simulink model "nonlinear_sim_FG"  (R2015a)
settings: Solver=ode45  StartTime=0.0  StopTime=100  RelTol=1e-3
values from neighbouring files (symbols this model uses):
  cbar = 3.45    [constants.m]
  g = 9.81    [constants.m]
  Iy = 75673.6    [constants.m]
  q_0 = 0    [constants.m]
  theta_0 = 0*(pi/180)    (= 0)    [constants.m]
  u_0 = 135    [constants.m]
  w_0 = 0    [constants.m]
  XE_0 = 0    [constants.m]    (also in controller_design.m)
  ZE_0 = -2000    [constants.m]    (also in controller_design.m)
  zt = 0.15    [constants.m]
undefined symbols (not defined in the file or in its folder): Earth, m, magnitude, WGS84
libraries: aerolibtransform2 x1, aerolibfltsims x1, vrlib x1
settings Model: Creator=vinay  LastModifiedBy=vinay

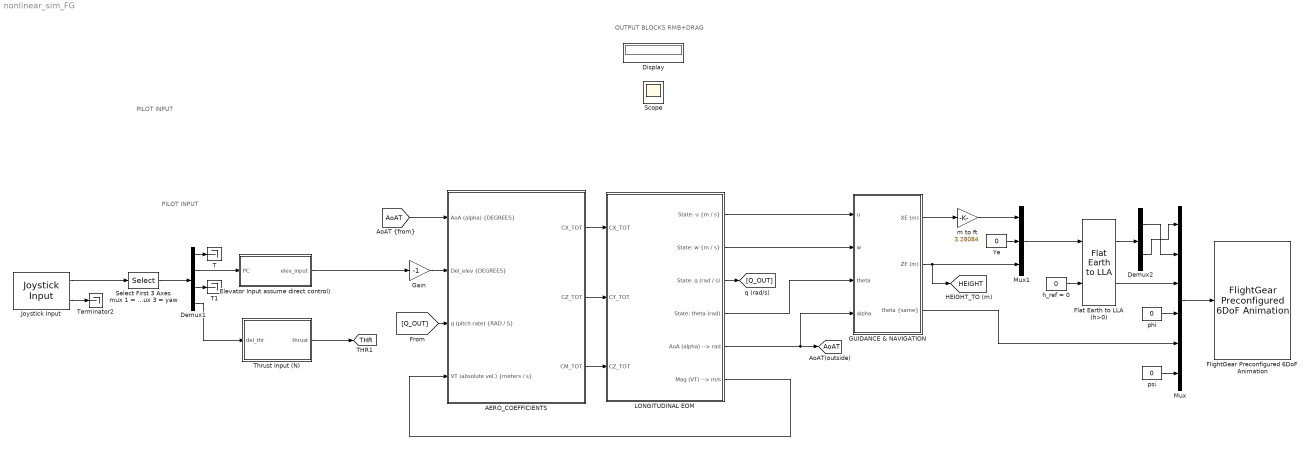
== system nonlinear_sim_FG ==
  note: PILOT INPUT
  note: OUTPUT BLOCKS
      | RMB+DRAG
  note: PILOT INPUT
  "AERO_COEFFICIENTS " : Subsystem
  Demux1 : Demux
  Demux2 : Demux  Outputs=2
  Display : Display
  Elevator Input assume direct control) : Subsystem
  Flat Earth to LLA (h>0) : aerolibtransform2/Flat Earth to LLA  units=Metric (MKS)  ptype=Earth (WGS84)  F=1/298.257223563  R=6378137  LL0=[34.8851654 -117.8323255]  psi=0
  FlightGear Preconfigured 6DoF Animation : aerolibfltsims/FlightGear Preconfigured 6DoF Animation  xFlightGearVersion=v3.0  DestinationIpAddress=127.0.0.1  DestinationPort=5502  SampleTime=1/30
  "GUIDANCE & NAVIGATION " : Subsystem
  Gain : Gain  Gain=-1
  Joystick Input : vrlib/Joystick Input  joyid=1  adjustports=off  forcefeed=off
  LONGITUDINAL EOM : Subsystem
  Mux : Mux  Inputs=6
  Mux1 : Mux  Inputs=3
  Scope : Scope
  Select First 3 Axes mux 1 = roll mux 2 = pitch mux 3 = yaw : Selector  InputPortWidth=8  Indices=[1 2 3 4]
      settings: AttributesFormatString=(Joystick - dependent)
  T : Terminator
  T1 : Terminator
  Terminator2 : Terminator
  Thrust Input (N) : Subsystem
  Ye : Constant  Value=0
  h_ref = 0 : Constant  Value=0
  m to ft : Gain  Gain=3.28084
  phi : Constant  Value=0
  psi : Constant  Value=0
  tag scope: AoAT=global, HEIGHT=global, THR=global
  wires:
  "AERO_COEFFICIENTS "/1(CX_TOT) -> LONGITUDINAL EOM/1(CX_TOT)
  "AERO_COEFFICIENTS "/2(CZ_TOT) -> LONGITUDINAL EOM/2(CY_TOT)
  "AERO_COEFFICIENTS "/3(CM_TOT) -> LONGITUDINAL EOM/3(CZ_TOT)
  [AoAT] -> "AERO_COEFFICIENTS "/1("AoA (alpha) {DEGREES}")
  LONGITUDINAL EOM/6(Mag (VT) --> m/s) -> "AERO_COEFFICIENTS "/4("VT (absolute vel.) {meters / s}")
  Elevator Input assume direct control)/1(elev_input) -> Gain/1
  LONGITUDINAL EOM/5(AoA (alpha) --> rad) -> [AoAT], "GUIDANCE & NAVIGATION "/4(alpha)
  LONGITUDINAL EOM/3(State: q (rad / s)) -> [Q_OUT]
  [Q_OUT] -> "AERO_COEFFICIENTS "/3("q (pitch rate) {RAD / S}")
  LONGITUDINAL EOM/1("State: u {m / s}") -> "GUIDANCE & NAVIGATION "/1(u)
  LONGITUDINAL EOM/2("State: w {m / s}") -> "GUIDANCE & NAVIGATION "/2(w)
  LONGITUDINAL EOM/4(State: theta (rad)) -> "GUIDANCE & NAVIGATION "/3(theta)
  "GUIDANCE & NAVIGATION "/2(ZE (m)) -> Mux1/3, [HEIGHT]
  Demux1/3 -> T1/1
  Select First 3 Axes mux 1 = roll mux 2 = pitch mux 3 = yaw/1 -> Demux1/1
  Demux1/2 -> Elevator Input assume direct control)/1(PC)
  Joystick Input/1 -> Select First 3 Axes mux 1 = roll mux 2 = pitch mux 3 = yaw/1
  Demux1/1 -> T/1
  Joystick Input/2 -> Terminator2/1
  Mux/1 -> FlightGear Preconfigured 6DoF Animation/1
  phi/1 -> Mux/4
  psi/1 -> Mux/6
  "GUIDANCE & NAVIGATION "/1(XE (m)) -> m to ft/1
  Ye/1 -> Mux1/2
  Mux1/1 -> Flat Earth to LLA (h>0)/1
  h_ref = 0/1 -> Flat Earth to LLA (h>0)/2
  Flat Earth to LLA (h>0)/1 -> Demux2/1
  Flat Earth to LLA (h>0)/2 -> Mux/3
  Demux2/1 -> Mux/2
  "GUIDANCE & NAVIGATION "/3("theta {same}") -> Mux/5
  Demux2/2 -> Mux/1
  Gain/1 -> "AERO_COEFFICIENTS "/2("Del_elev {DEGREES}")
  Demux1/4 -> Thrust Input (N)/1(del_thr)
  Thrust Input (N)/1(thrust) -> [THR]
  m to ft/1 -> Mux1/1

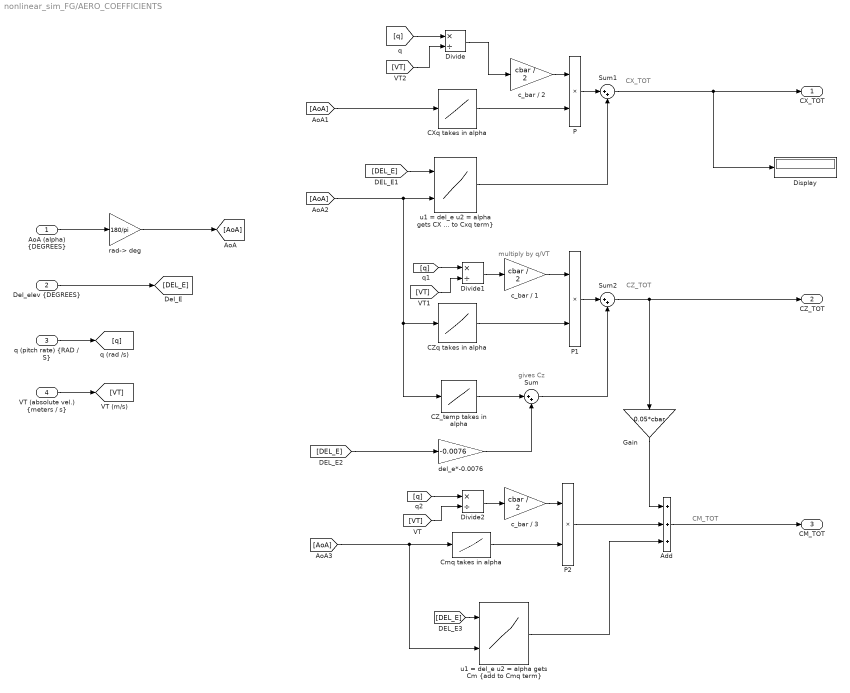
== system nonlinear_sim_FG/AERO_COEFFICIENTS  ==
  note: multiply by q/VT
  note: CM_TOT
  note: CX_TOT
  note: gives Cz
  note: CZ_TOT
  "AoA (alpha) {DEGREES}" : Inport
  "Del_elev {DEGREES}" : Inport  Port=2
  "q (pitch rate) {RAD / S}" : Inport  Port=3
  "VT (absolute vel.) {meters / s}" : Inport  Port=4
  Add : Sum  Inputs=+++
  CXq takes in alpha : Lookup_n-D  NumberOfTableDimensions=1  BreakpointsForDimension1=[-10,-5,0,5,10,15,20,25,30,35,40,45]  BreakpointsForDimension1Min=[-10]  BreakpointsForDimension1Max=[10]  Table=[-.267,.110,.308,1.34,2.08,2.91,2.76,2.05,1.5,1.49,1.83,1.21]  InternalRulePriority=Speed  OutMin=[-1.000]  OutMax=[1.000]  RndMeth=Simplest  InputSameDT=on
  CZ_temp takes in alpha : Lookup_n-D  NumberOfTableDimensions=1  BreakpointsForDimension1=[-10,-5,0,5,10,15,20,25,30,35,40,45]  BreakpointsForDimension1Min=[-10]  BreakpointsForDimension1Max=[10]  Table=[.770, .241, -.100, -.416, -.731, -1.053, -1.366, -1.646, -1.917, -2.120, -2.248, -2.229]  InternalRulePriority=Speed  OutMin=[-1.000]  OutMax=[1.000]  RndMeth=Simplest  InputSameDT=on
  CZq takes in alpha : Lookup_n-D  NumberOfTableDimensions=1  BreakpointsForDimension1=[-10,-5,0,5,10,15,20,25,30,35,40,45]  BreakpointsForDimension1Min=[-10]  BreakpointsForDimension1Max=[10]  Table="[-8.8, -25.8, -28.9, -31.4, -31.2, -30.7, -27.7, -28.2,   -29, -29.8, -38.3, -35.3]"  InternalRulePriority=Speed  OutMin=[-1.000]  OutMax=[1.000]  RndMeth=Simplest  InputSameDT=on
  Cmq takes in alpha : Lookup_n-D  NumberOfTableDimensions=1  BreakpointsForDimension1=[-10,-5,0,5,10,15,20,25,30,35,40,45]  BreakpointsForDimension1Min=[-10]  BreakpointsForDimension1Max=[10]  Table="[-7.21,  -.54, -5.23, -5.26, -6.11, -6.64, -5.69,    -6,  -6.2,  -6.4,  -6.6,    -6]"  InternalRulePriority=Speed  OutMin=[-1.000]  OutMax=[1.000]  RndMeth=Simplest  InputSameDT=on
  Display : Display
  Divide : Product  Inputs=*/
  Divide1 : Product  Inputs=*/
  Divide2 : Product  Inputs=*/
  Gain : Gain  Gain=0.05*cbar
  P : Product
  P1 : Product
  P2 : Product
  Sum : Sum  Inputs=|++
  Sum1 : Sum  Inputs=|++
  Sum2 : Sum  Inputs=|++
  c_bar / 1 : Gain  Gain=cbar / 2
  c_bar / 2 : Gain  Gain=cbar / 2
  c_bar / 3 : Gain  Gain=cbar / 2
  del_e*-0.0076 : Gain  Gain=-0.0076
  rad-> deg : Gain  Gain=180/pi
  "u1 = del_e u2 = alpha gets CX {add to Cxq term}" : Lookup_n-D  BreakpointsForDimension1=[-25 -12.5 0 12.5 25]  BreakpointsForDimension2=[-10 -5 0 5 10 15 20 25 30 35 40 45]  IndexSearchMethod=Evenly spaced points  Table="[-.083, -.073, -.076, -.072, -.046, .012, .024, .025, .043, .053, .047, .040; -.040, -.038, -.039, -.025,  .006, .062, .087, .085, .100, .110, .104, .091;-.022, -.020, -.021, -.004,  .032, .094, .128, .130, .154, .161, .155, .138; -.048, -.038, -.040, -.021,  .016, .083, .127, .137, .162, .177, .179, .167; -.099, -.081, -.081, -.063, -.025, .044, .097, .113, .145, .167, .174, .166]"  InternalRulePriority=Speed  RndMeth=Simplest  InputSameDT=on
  "u1 = del_e u2 = alpha gets Cm {add to Cmq term}" : Lookup_n-D  BreakpointsForDimension1=[-25 -12.5 0 12.5 25]  BreakpointsForDimension2=[-10 -5 0 5 10 15 20 25 30 35 40 45]  IndexSearchMethod=Evenly spaced points  Table="[.205,  .168,  .186,  .196,  .213,  .251,  .245,  .238,  .252,  .231,  .198,  .192; .081,  .077,  .107,  .110,  .110,  .141,  .127,  .119,  .133,  .108,  .081,  .093; -.046, -.020, -.009, -.005, -.006,  .010,  .006, -.001,  .014,   0.0, -.013,  .032; -.174, -.145, -.121, -.127, -.129, -.102, -.097, -.113, -.087, -.084, -.069, -.006; -.259, -.202, -.184, -.193, -.199, -.150, -.160, -.167, -.104, -.076, -.041, -.005]"  InternalRulePriority=Speed  RndMeth=Simplest  InputSameDT=on
  CX_TOT : Outport
  CZ_TOT : Outport  Port=2
  CM_TOT : Outport  Port=3
  wires:
  P2/1 -> Add/2
  "q (pitch rate) {RAD / S}"/1 -> [q]
  Cmq takes in alpha/1 -> P2/2
  Divide2/1 -> c_bar / 3/1
  Add/1 -> CM_TOT/1
  [VT] -> Divide/2
  P1/1 -> Sum2/1
  Sum/1 -> Sum2/2
  CZq takes in alpha/1 -> P1/2
  c_bar / 1/1 -> P1/1
  Sum2/1 -> CZ_TOT/1, Gain/1
  [VT] -> Divide1/2
  del_e*-0.0076/1 -> Sum/2
  CZ_temp takes in alpha/1 -> Sum/1
  P/1 -> Sum1/1
  c_bar / 3/1 -> P2/1
  "u1 = del_e u2 = alpha gets Cm {add to Cmq term}"/1 -> Add/3
  [q] -> Divide1/1
  [DEL_E] -> "u1 = del_e u2 = alpha gets Cm {add to Cmq term}"/1
  "u1 = del_e u2 = alpha gets CX {add to Cxq term}"/1 -> Sum1/2
  CXq takes in alpha/1 -> P/2
  Sum1/1 -> Display/1, CX_TOT/1
  c_bar / 2/1 -> P/1
  "VT (absolute vel.) {meters / s}"/1 -> [VT]
  [DEL_E] -> del_e*-0.0076/1
  [AoA] -> "u1 = del_e u2 = alpha gets CX {add to Cxq term}"/2, CZ_temp takes in alpha/1, CZq takes in alpha/1
  [DEL_E] -> "u1 = del_e u2 = alpha gets CX {add to Cxq term}"/1
  Gain/1 -> Add/1
  "AoA (alpha) {DEGREES}"/1 -> rad-> deg/1
  Divide1/1 -> c_bar / 1/1
  [AoA] -> "u1 = del_e u2 = alpha gets Cm {add to Cmq term}"/2, Cmq takes in alpha/1
  [q] -> Divide/1
  [VT] -> Divide2/2
  Divide/1 -> c_bar / 2/1
  [q] -> Divide2/1
  [AoA] -> CXq takes in alpha/1
  rad-> deg/1 -> [AoA]
  "Del_elev {DEGREES}"/1 -> [DEL_E]

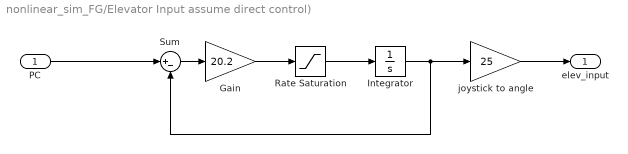
== system nonlinear_sim_FG/Elevator Input assume direct control) ==
  PC : Inport
  Gain : Gain  Gain=20.2  SaturateOnIntegerOverflow=on  OutDataTypeStr=Inherit: Same as input  ParamDataTypeStr=Inherit: Same as input
  "Integrator " : Integrator  InitialCondition=-2.4607  UpperSaturationLimit=25  LowerSaturationLimit=-25
  Rate Saturation : Saturate  UpperLimit=60  LowerLimit=-60
  Sum : Sum  Inputs=|+-  SaturateOnIntegerOverflow=on  InputSameDT=on  OutDataTypeStr=Inherit: Same as first input
  joystick to angle : Gain  Gain=25  SaturateOnIntegerOverflow=on  OutDataTypeStr=Inherit: Same as input  ParamDataTypeStr=Inherit: Same as input
  elev_input : Outport
  wires:
  PC/1 -> Sum/1
  Sum/1 -> Gain/1
  Gain/1 -> Rate Saturation/1
  Rate Saturation/1 -> "Integrator "/1
  "Integrator "/1 -> joystick to angle/1, Sum/2
  joystick to angle/1 -> elev_input/1

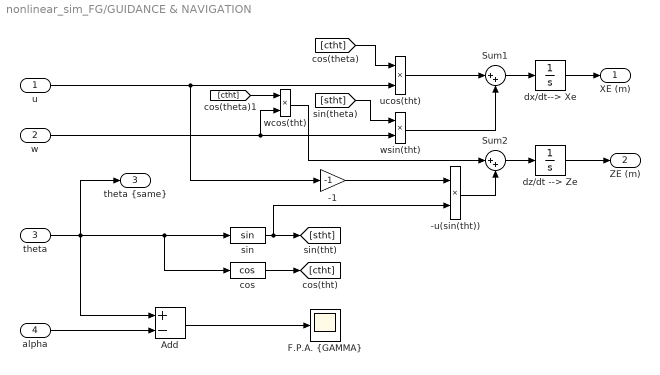
== system nonlinear_sim_FG/GUIDANCE & NAVIGATION  ==
  u : Inport
  w : Inport  Port=2
  theta : Inport  Port=3
  alpha : Inport  Port=4
  -1 : Gain  Gain=-1
  -u(sin(tht)) : Product
  Add : Sum  Inputs=+-
  "F.P.A. {GAMMA}" : Scope
      settings: SaveName=ScopeData2
  Sum1 : Sum  Inputs=|++
  Sum2 : Sum  Inputs=|++
  cos : Trigonometry  Operator=cos
  dx/dt--> Xe : Integrator  InitialCondition=XE_0
  dz/dt --> Ze : Integrator  InitialCondition=ZE_0
  sin : Trigonometry
  ucos(tht) : Product
  wcos(tht) : Product
  wsin(tht) : Product
  XE (m) : Outport
  ZE (m) : Outport  Port=2
  "theta {same}" : Outport  Port=3
  wires:
  [stht] -> wsin(tht)/1
  wsin(tht)/1 -> Sum1/2
  u/1 -> ucos(tht)/2, -1/1
  w/1 -> wcos(tht)/2, wsin(tht)/2
  theta/1 -> "theta {same}"/1, Add/1, cos/1, sin/1
  dx/dt--> Xe/1 -> XE (m)/1
  ucos(tht)/1 -> Sum1/1
  dz/dt --> Ze/1 -> ZE (m)/1
  Sum1/1 -> dx/dt--> Xe/1
  Sum2/1 -> dz/dt --> Ze/1
  cos/1 -> [ctht]
  sin/1 -> -u(sin(tht))/2, [stht]
  wcos(tht)/1 -> Sum2/1
  [ctht] -> wcos(tht)/1
  -1/1 -> -u(sin(tht))/1
  [ctht] -> ucos(tht)/1
  -u(sin(tht))/1 -> Sum2/2
  alpha/1 -> Add/2
  Add/1 -> "F.P.A. {GAMMA}"/1

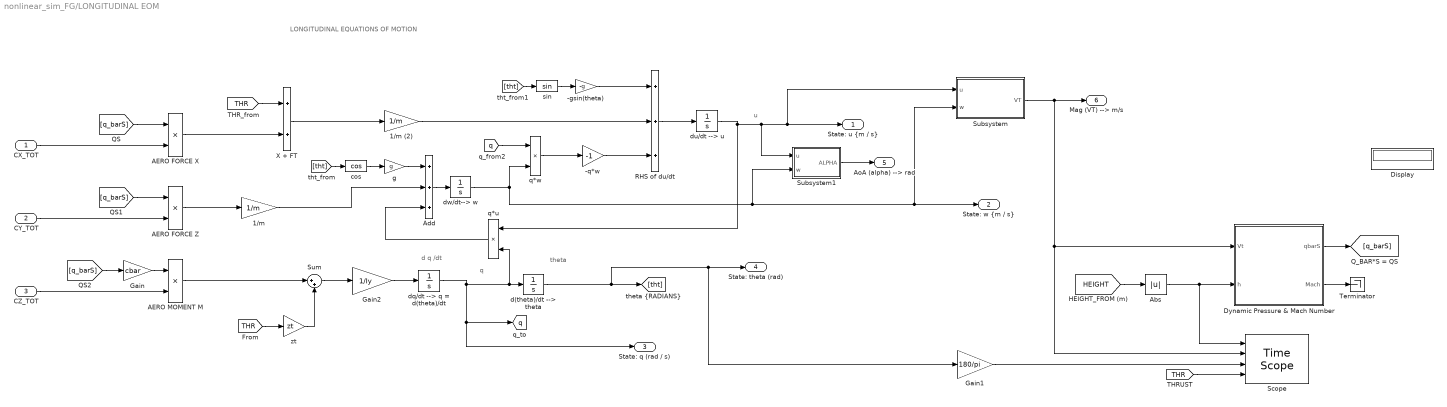
== system nonlinear_sim_FG/LONGITUDINAL EOM ==
  note: LONGITUDINAL EQUATIONS OF MOTION
  note: u
  note: theta
  note: q
  note: d q /dt
  CX_TOT : Inport
  CY_TOT : Inport  Port=2
  CZ_TOT : Inport  Port=3
  -gsin(theta) : Gain  Gain=-g
  -q*w : Gain  Gain=-1
  1/m : Gain  Gain=1/m
  1/m (2) : Gain  Gain=1/m
  AERO FORCE X : Product
  AERO FORCE Z : Product
  AERO MOMENT M : Product
  Abs : Abs
  Add : Sum  Inputs=+++
  Display : Display
  Dynamic Pressure & Mach Number : MATLAB Function  TreatAsAtomicUnit=on
  Gain : Gain  Gain=cbar
  Gain1 : Gain  Gain=180/pi
  Gain2 : Gain  Gain=1/Iy
  RHS of du/dt : Sum  Inputs=+++
  Scope : TimeScope  NumInputPorts=4
  Subsystem : Subsystem
  Subsystem1 : Subsystem
  Sum : Sum  Inputs=|++
  Terminator : Terminator
  X + FT : Sum
  cos : Trigonometry  Operator=cos
  d(theta)/dt --> theta : Integrator  InitialCondition=theta_0
  dq/dt --> q = d(theta)/dt : Integrator  InitialCondition=q_0
  du/dt --> u : Integrator  InitialCondition=u_0  LimitOutput=on  LowerSaturationLimit=0
  dw/dt--> w : Integrator  InitialCondition=w_0
  g : Gain  Gain=g
  q*u : Product
  q*w : Product
  sin : Trigonometry
  zt : Gain  Gain=zt
  "State: u {m / s}" : Outport
  "State: w {m / s}" : Outport  Port=2
  State: q (rad / s) : Outport  Port=3
  State: theta (rad) : Outport  Port=4
  AoA (alpha) --> rad : Outport  Port=5
  Mag (VT) --> m/s : Outport  Port=6
  tag scope: q=global
  wires:
  [THR] -> X + FT/1
  q*w/1 -> -q*w/1
  zt/1 -> Sum/2
  Gain2/1 -> dq/dt --> q = d(theta)/dt/1
  dq/dt --> q = d(theta)/dt/1 -> State: q (rad / s)/1, [q], q*u/2, d(theta)/dt --> theta/1
  -gsin(theta)/1 -> RHS of du/dt/1
  [q] -> q*w/1
  1/m/1 -> Add/2
  AERO FORCE X/1 -> X + FT/2
  AERO MOMENT M/1 -> Sum/1
  [THR] -> zt/1
  [tht] -> sin/1
  sin/1 -> -gsin(theta)/1
  CY_TOT/1 -> AERO FORCE Z/2
  [q_barS] -> AERO FORCE Z/1
  CX_TOT/1 -> AERO FORCE X/2
  [q_barS] -> AERO FORCE X/1
  CZ_TOT/1 -> AERO MOMENT M/2
  [q_barS] -> Gain/1
  Gain/1 -> AERO MOMENT M/1
  d(theta)/dt --> theta/1 -> Gain1/1, State: theta (rad)/1, [tht]
  Sum/1 -> Gain2/1
  AERO FORCE Z/1 -> 1/m/1
  g/1 -> Add/1
  Add/1 -> dw/dt--> w/1
  cos/1 -> g/1
  q*u/1 -> Add/3
  [tht] -> cos/1
  RHS of du/dt/1 -> du/dt --> u/1
  1/m (2)/1 -> RHS of du/dt/2
  X + FT/1 -> 1/m (2)/1
  -q*w/1 -> RHS of du/dt/3
  du/dt --> u/1 -> Subsystem1/1(u), Subsystem/1(u), "State: u {m / s}"/1, q*u/1
  dw/dt--> w/1 -> Subsystem1/2(w), Subsystem/2(w), "State: w {m / s}"/1, q*w/2
  Dynamic Pressure & Mach Number/1(qbarS) -> [q_barS]
  [HEIGHT] -> Abs/1
  Dynamic Pressure & Mach Number/2(Mach) -> Terminator/1
  Subsystem/1(VT) -> Scope/2, Dynamic Pressure & Mach Number/1(Vt), Mag (VT) --> m/s/1
  Subsystem1/1(ALPHA) -> AoA (alpha) --> rad/1
  Abs/1 -> Scope/1, Dynamic Pressure & Mach Number/2(h)
  Gain1/1 -> Scope/3
  [THR] -> Scope/4

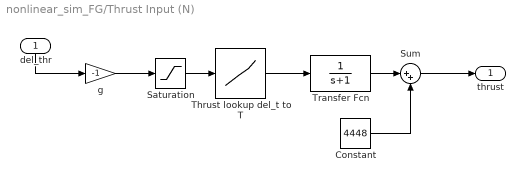
== system nonlinear_sim_FG/Thrust Input (N) ==
  del_thr : Inport
  Constant : Constant  Value=4448
  Saturation : Saturate  UpperLimit=0.75  LowerLimit=0.15
  Sum : Sum  Inputs=|++
  Thrust lookup del_t to T : Lookup_n-D  NumberOfTableDimensions=1  BreakpointsForDimension1=[0.15000, .19470, .23950, .28420, .32890, .37370, .41840, .4632, 0.5079, 0.5526, 0.5974, 0.6421, 0.6868, 0.7316, 0.7763, 0.8211, 0.8658, 0.9105, 0.9553, 1.0000]  Table=[4448.00, 8662.11, 12876.21, 17090.32, 21304.42 , 25518.53, 29732.63, 33946.74, 38160.84, 42374.95, 46589.05, 50803.16, 55017.26, 59231.37, 63445.47, 67659.58, 71873.6, 76087.7, 80301.89, 84516.00]  InternalRulePriority=Speed  RndMeth=Simplest  InputSameDT=on
  Transfer Fcn : TransferFcn  Denominator=[1 1]
  g : Gain  Gain=-1
  thrust : Outport
  wires:
  del_thr/1 -> g/1
  Saturation/1 -> Thrust lookup del_t to T/1
  g/1 -> Saturation/1
  Thrust lookup del_t to T/1 -> Transfer Fcn/1
  Transfer Fcn/1 -> Sum/1
  Sum/1 -> thrust/1
  Constant/1 -> Sum/2

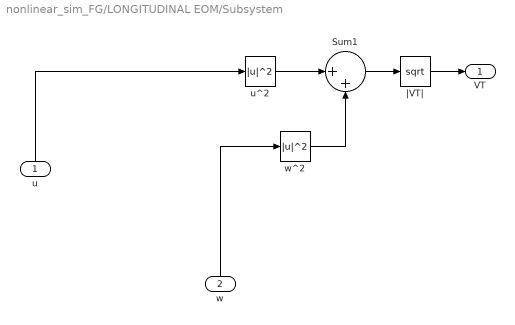
== system nonlinear_sim_FG/LONGITUDINAL EOM/Subsystem ==
  u : Inport
  w : Inport  Port=2
  Sum1 : Sum  Inputs=|++
  u^2 : Math  Operator=magnitude^2  SaturateOnIntegerOverflow=on
  w^2 : Math  Operator=magnitude^2  SaturateOnIntegerOverflow=on
  |VT| : Sqrt  SaturateOnIntegerOverflow=on
  VT : Outport
  wires:
  Sum1/1 -> |VT|/1
  |VT|/1 -> VT/1
  u^2/1 -> Sum1/1
  w^2/1 -> Sum1/2
  w/1 -> w^2/1
  u/1 -> u^2/1

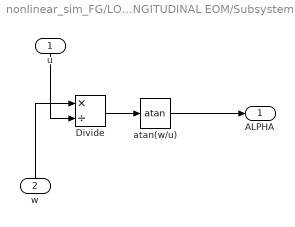
== system nonlinear_sim_FG/LONGITUDINAL EOM/Subsystem1 ==
  u : Inport
  w : Inport  Port=2
  Divide : Product  Inputs=*/
  atan(w/u) : Trigonometry  Operator=atan
  ALPHA : Outport
  wires:
  Divide/1 -> atan(w/u)/1
  w/1 -> Divide/1
  u/1 -> Divide/2
  atan(w/u)/1 -> ALPHA/1

== matlab function nonlinear_sim_FG/LONGITUDINAL EOM/Dynamic Pressure & Mach Number ==
  data: Vt input; qbarS output; h input; Mach output
function [qbarS, Mach] = ATMOS(Vt, h)
%#codegen
%SI UNITS EVERYTHING
%calculate density
%max height, note h > 0
if h>=11000
    h = 11000;
end
T = 288.15 - 0.0065*h;
rho = 1.225*exp(-9.81*h/(287.05*T));
a = sqrt(1.4*287.05*T);

%dynamic pressure
q_bar = 0.5*Vt^2*rho;
S = 27.87;

%Mach #
Mach = Vt/a;
qbarS = q_bar*S;
